simulink subsystem "OdometriaZ"  (R2023b)
settings: Solver=VariableStepAuto  StartTime=0.0  StopTime=10.0  RelTol=1e-3
undefined symbols (not defined in the file): DiscIntNeverNeededParam
settings Model: Creator=USUARIO  LastModifiedBy=USUARIO

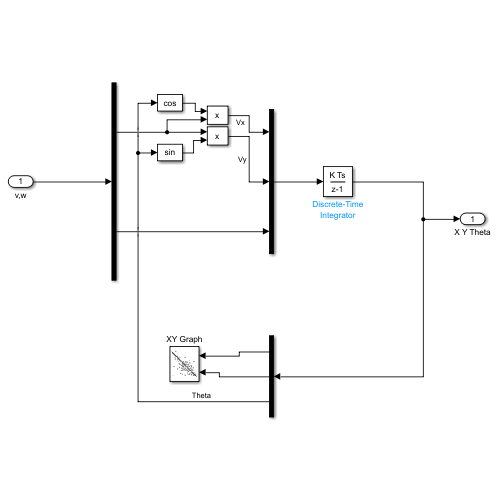
[thumbnail: Simulink's stored preview of the top-level diagram]
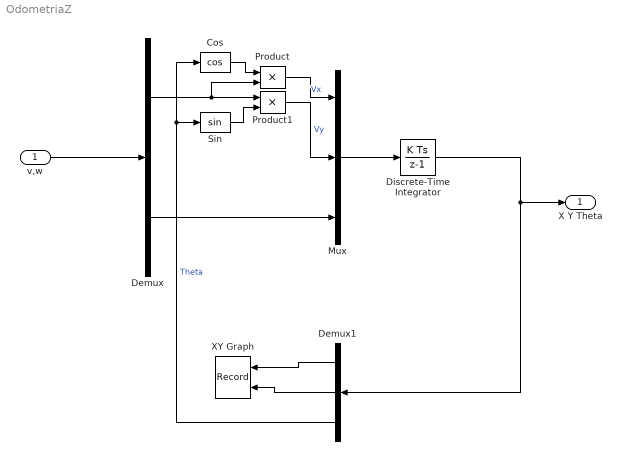
== system OdometriaZ ==
  v,w : Inport
  Cos : Trigonometry  Operator=cos
  Demux : Demux  Outputs=2
  Demux1 : Demux  Outputs=3
  Discrete-Time Integrator : DiscreteIntegrator  SampleTime=-1  ICPrevOutput=DiscIntNeverNeededParam  ICPrevScaledInput=DiscIntNeverNeededParam
  Mux : Mux  Inputs=3
  Product : Product
  Product1 : Product
  Sin : Trigonometry
  XY Graph : Record  FileSettingsInternal="{\"entries\":[{\"content\":{\"excelSettings\":{\"content\":{},\"type\":\"Streamout.ExcelSettings\"}},\"type\":\"Streamout.FileSettingStorage\",\"uuid\":\"\"}],\"packageUris\":[\"http:\\/\\/schema.mathworks.com\\/mf0\\/streamout_blocks\\/R2020a\"],\"version\":\"1.0\"}"  Layout=[1 1]  SignalsInternal="{\"entries\":[{\"content\":{\"signals\":[{\"content\":{\"blockPath\":[],\"dimensions\":[1],\"domain\":\"\",\"lineColor\":\"#a2142f\",\"plots\":[1],\"port\":1,\"signalID\":119,\"signalName\":\"Demux1:1\"},\"type\":\"RecordBlkView.Signal\",\"uuid\":\"\"},{\"content\":{\"blockPath\":[],\"dimensions\":[1],\"domain\":\"\",\"lineColor\":\"#139fff\",\"plots\":[1],\"port\":2,\"signalID\":122,\"signalName\":\"Demux1:2\"},\"type\":\"RecordBlkView.Signal\",\"uuid\":\"\"}]},\"type\":\"RecordBlkView.InputSignals\",\"uuid\":\"\"}],\"packageUris\":[\"http:\\/\\/schema.mathworks.com\\/mf0\\/streamout_blocks\\/R2020a\"],\"version\":\"1.0\"}"  VisualizationBindings="{\"xyplotplugin\":{\"info\":[{\"series\":[{\"bindingParametersList\":[{\"parameter\":\"X-Axis\",\"signalID\":119,\"signalName\":\"Demux1:1\"},{\"parameter\":\"Y-Axis\",\"signalID\":122,\"signalName\":\"Demux1:2\"}],\"seriesID\":42512}],\"subplotID\":1}]}}"  CompatibilityTag=XY
  X Y Theta : Outport
  wires:
  Demux1/2 -> XY Graph/2
  Demux1/1 -> XY Graph/1
  Mux/1 -> Discrete-Time Integrator/1
  Discrete-Time Integrator/1 -> Demux1/1, X Y Theta/1
  Product1/1 -> Mux/2  "Vy"
  Demux/1 -> Product/2, Product1/1
  Product/1 -> Mux/1  "Vx"
  v,w/1 -> Demux/1
  Demux1/3 -> Cos/1, Sin/1  "Theta"
  Demux/2 -> Mux/3
  Sin/1 -> Product1/2
  Cos/1 -> Product/1
